simulink model "SiDLEngine"  (R2021a)
settings: Solver=VariableStepAuto  StartTime=0.0  StopTime=inf  FixedStep=0.03  RelTol=1e-3  EnableMultiTasking=on
model workspace (MAT data in the model file):
  AfrStoich = 14.6
  Cps = 2
  FuelSg = 0.75
  NCyl = 4
  Pstd = 101325
  Rair = 287
  TimeCnstECP = 0.01
  TimeCnstEGR = 0.01
  TimeCnstETC = 0.01
  TimeCnstICP = 0.01
  TimeCnstIVL = 0.125
  TimeCnstMFA = 0.125
  TimeCnstSWVA = 0.125
  TimeCnstVCR = 0.125
  TimeCnstVGT = 0.15
  TimeCnstVIRL = 0.125
  TimeCnstWGA = 0.01
  Ts = 0.01
  Tstd = 293.15
  Vd = 0.0015
  layer2Bias = [-0.102818198502 -0.0669189542532 -0.0175336152315 -0.0613032355905 -0.0570961982012 -0.061625469476 -0.0630445405841 -0.102546460927 -0.0423759259284 -0.0306564457715 -0.0652378797531 -0.129787817597 ... (800 elements, 800x1)]
  layer2InputWeights = [-0.0867959260941 0.0265881456435 -0.00261938013136 0.0648385435343 -0.0334306880832 -0.044301789254 0.0604524612427 0.00893297791481 -0.0994751527905 0.0255589019507 -0.122370123863 -0.0740034654737 ... (1600 elements, 800x2)]
  layer2RecurrentWeights = [-0.015235141851 -0.11403311789 0.112884886563 0.0588350631297 0.0682250186801 0.0444636531174 -0.0968889594078 -0.0397337339818 -0.0227067749947 0.0294026453048 -0.0304179247469 -0.145884677768 ... (160000 elements, 800x200)]
  layer3Bias = [0.0529259070754; 0.0636636316776; 0.0140457563102; 0.0780845806003; 0.0347621031106; -0.023198319599; -0.0368600413203; -0.00711429771036; -0.0257519558072; 0.0254531633109; 0.0144603000954]
  layer3Weights = [0.0566984564066 0.0242331400514 0.158808469772 0.0399505831301 -0.0030719502829 0.0837587192655 0.0579013302922 -0.0333247296512 -0.120384372771 -0.125806882977 0.0938690528274 -0.052338026464 ... (2200 elements, 11x200)]
  muX = [2220.83734119 107.92815484]
  muY = [104.671657967 115562.072489 0.00224719893222 986.056400633 7383.06398882 0.0299760704621 325.741103054 5.88867806863e-05 0.000942478781448 3.56158507349e-05 0.00543639293543]
  sigX = [1470.27383875 63.5647381428]
  sigY = [65.6275263528 46686.4071583 0.00207427504126 224.539922164 5111.0011239 0.0252132241042 8.06209455442 0.000125926264941 0.00171123843744 4.89959895827e-05 0.00480295587248]
libraries: autolibutils x4, simulink x2, autolibsharedmappedenginescommon x1, autolibpowerinfoutils x1
(part 1 of 2)
settings Model: ModifiedByFormat=The MathWorks, Inc.  OrderedModelArguments=off  Creator=The MathWorks, Inc.  LastModifiedBy=The MathWorks, Inc.
settings SolverCC: AlgebraicLoopSolver=TrustRegion  DecoupledContinuousIntegration=on
settings DataIOCC: DSMLogging=off  ReturnWorkspaceOutputs=off
settings DebuggingCC: SFMachineParentedDataDiag=warning  ArithmeticOperatorsInVariantConditions=warning
settings SFSimCC: SimUseLocalCustomCode=off
settings RTWCC: RTWUseLocalCustomCode=off
settings CodeAppCC: StateflowObjectComments=on
settings GRTTargetCC: TargetLangStandard=C89/C90 (ANSI)
settings ConfigComp: CovMetricSettings=dsw  CovSaveCumulativeToWorkspaceVar=on  CovSaveSingleToWorkspaceVar=on  CovExternalEMLEnable=off
settings SimscapeCC: SimscapeNormalizeSystem=off  SimscapeNominalValues={1, 'bar'; 1, 'cm^3/s'; 1, 'bar*kg/s'; 1, 'kJ/kg'; 1, 'kW'}

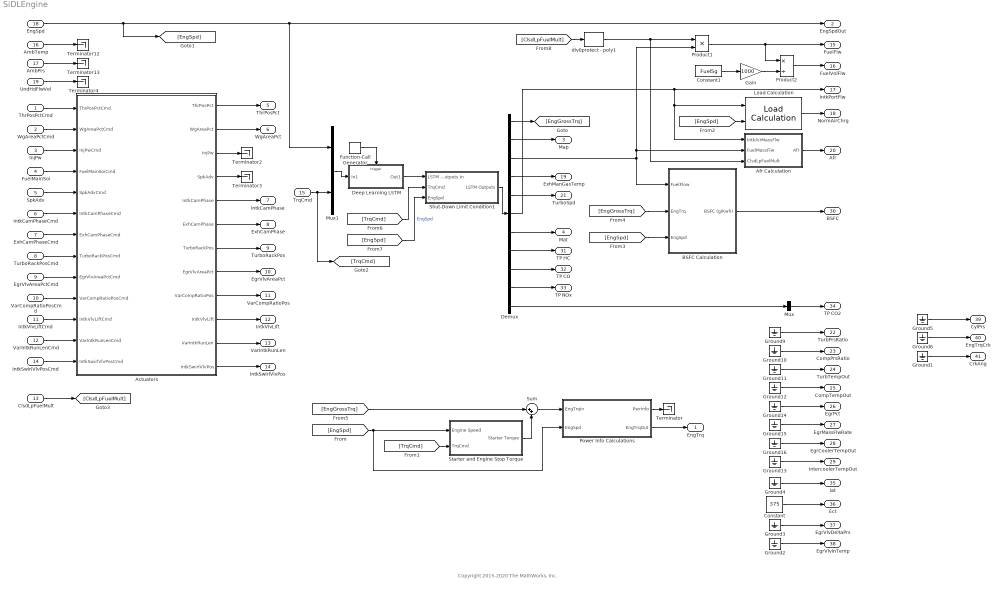
== system SiDLEngine ==
  note: Copyright 2015-2020 The MathWorks, Inc.
  ThrPosPctCmd : Inport
  WgAreaPctCmd : Inport  Port=2
  InjPw : Inport  Port=3
  FuelMainSoi : Inport  Port=4
  SpkAdv : Inport  Port=5
  IntkCamPhaseCmd : Inport  Port=6
  ExhCamPhaseCmd : Inport  Port=7
  TurboRackPosCmd : Inport  Port=8
  EgrVlvAreaPctCmd : Inport  Port=9
  VarCompRatioPosCmd : Inport  Port=10
  IntkVlvLiftCmd : Inport  Port=11
  VarIntkRunLenCmd : Inport  Port=12
  ClsdLpFuelMult : Inport  Port=13  Unit=1
  IntkSwirlVlvPosCmd : Inport  Port=14
  TrqCmd : Inport  Port=15  Unit=N*m
  AmbTemp : Inport  Port=16  Unit=K
  AmbPrs : Inport  Port=17  Unit=Pa
  EngSpd : Inport  Port=18  Interpolate=off
  UndHdFlwVel : Inport  Port=19  Unit=m/s
  Actuators : Subsystem
  Afr Calculation : Subsystem
  BSFC Calculation : Subsystem
  Constant : Constant  Value=375
  Constant1 : Constant  Value=FuelSg
  Deep Learning LSTM : Subsystem  TreatAsAtomicUnit=on
  Demux : Demux  Outputs=11
  Function-Call Generator : simulink/Ports & Subsystems/Function-Call Generator  sample_time=Ts  numberOfIterations=1  DisallowWideOutput=off
  Gain : Gain  Gain=1000
  Ground{1..6,9..16} (14 alike) : Ground
  Load Calculation : autolibsharedmappedenginescommon/Load Calculation  SystemSampleTime=-1  VariantActivationTime=update diagram  Latency=0  AutoFrameSizeCalculation=off
      settings: SourceProductBaseCode=PW,DR,MT,UV,VE
  Mux : Mux  Inputs=1
  Mux1 : Mux  Inputs=2
  Power Info Calculations : Subsystem
  Product1 : Product
  Product2 : Product  Inputs=*/
  Shut-Down Limit Condition1 : Subsystem
  Starter and Engine Stop Torque : Subsystem
  Sum : Sum  Inputs=|++
  Terminator{,2..4,12..13} (6 alike) : Terminator
  div0protect - poly1 : autolibutils/div0protect - poly  thresh=0.01  ZeroCross1=off  aMode=aMode
      settings: SourceProductBaseCode=PW,DR,MT,UV,VE
  EngTrq : Outport  Unit=N*m  VectorParamsAs1DForOutWhenUnconnected=off
  EngSpdOut : Outport  Port=2  VectorParamsAs1DForOutWhenUnconnected=off
  Map : Outport  Port=3  Unit=Pa  VectorParamsAs1DForOutWhenUnconnected=off
  Mat : Outport  Port=4  Unit=K  VectorParamsAs1DForOutWhenUnconnected=off
  ThrPosPct : Outport  Port=5  VectorParamsAs1DForOutWhenUnconnected=off
  WgAreaPct : Outport  Port=6  VectorParamsAs1DForOutWhenUnconnected=off
  IntkCamPhase : Outport  Port=7  VectorParamsAs1DForOutWhenUnconnected=off
  ExhCamPhase : Outport  Port=8  VectorParamsAs1DForOutWhenUnconnected=off
  TurboRackPos : Outport  Port=9  VectorParamsAs1DForOutWhenUnconnected=off
  EgrVlvAreaPct : Outport  Port=10  VectorParamsAs1DForOutWhenUnconnected=off
  VarCompRatioPos : Outport  Port=11  VectorParamsAs1DForOutWhenUnconnected=off
  IntkVlvLift : Outport  Port=12  VectorParamsAs1DForOutWhenUnconnected=off
  VarIntkRunLen : Outport  Port=13  VectorParamsAs1DForOutWhenUnconnected=off
  IntkSwirlVlvPos : Outport  Port=14  VectorParamsAs1DForOutWhenUnconnected=off
  FuelFlw : Outport  Port=15  Unit=kg/s  VectorParamsAs1DForOutWhenUnconnected=off
  FuelVolFlw : Outport  Port=16  Unit=m^3/s  VectorParamsAs1DForOutWhenUnconnected=off
  IntkPortFlw : Outport  Port=17  Unit=kg/s  VectorParamsAs1DForOutWhenUnconnected=off
  NormAirChrg : Outport  Port=18  Unit=1  VectorParamsAs1DForOutWhenUnconnected=off
  ExhManGasTemp : Outport  Port=19  Unit=K  VectorParamsAs1DForOutWhenUnconnected=off
  Afr : Outport  Port=20  Unit=1  VectorParamsAs1DForOutWhenUnconnected=off
  TurboSpd : Outport  Port=21  Unit=rad/s  VectorParamsAs1DForOutWhenUnconnected=off
  TurbPrsRatio : Outport  Port=22  Unit=1  VectorParamsAs1DForOutWhenUnconnected=off
  CompPrsRatio : Outport  Port=23  Unit=1  VectorParamsAs1DForOutWhenUnconnected=off
  TurbTempOut : Outport  Port=24  Unit=K  VectorParamsAs1DForOutWhenUnconnected=off
  CompTempOut : Outport  Port=25  Unit=K  VectorParamsAs1DForOutWhenUnconnected=off
  EgrPct : Outport  Port=26  Unit=%  VectorParamsAs1DForOutWhenUnconnected=off
  EgrMassFlwRate : Outport  Port=27  Unit=kg/s  VectorParamsAs1DForOutWhenUnconnected=off
  EgrCoolerTempOut : Outport  Port=28  Unit=K  VectorParamsAs1DForOutWhenUnconnected=off
  IntercoolerTempOut : Outport  Port=29  Unit=K  VectorParamsAs1DForOutWhenUnconnected=off
  BSFC : Outport  Port=30  Unit=g/(kW*hr)  VectorParamsAs1DForOutWhenUnconnected=off
  TP HC : Outport  Port=31  Unit=kg/s  VectorParamsAs1DForOutWhenUnconnected=off
  TP CO : Outport  Port=32  Unit=kg/s  VectorParamsAs1DForOutWhenUnconnected=off
  TP NOx : Outport  Port=33  Unit=kg/s  VectorParamsAs1DForOutWhenUnconnected=off
  TP CO2 : Outport  Port=34  Unit=kg/s  VectorParamsAs1DForOutWhenUnconnected=off
  Iat : Outport  Port=35  Unit=K  VectorParamsAs1DForOutWhenUnconnected=off
  Ect : Outport  Port=36  Unit=K  VectorParamsAs1DForOutWhenUnconnected=off
  EgrVlvDeltaPrs : Outport  Port=37  Unit=Pa  VectorParamsAs1DForOutWhenUnconnected=off
  EgrVlvInTemp : Outport  Port=38  Unit=K  VectorParamsAs1DForOutWhenUnconnected=off
  CylPrs : Outport  Port=39  VectorParamsAs1DForOutWhenUnconnected=off
  EngTrqCrk : Outport  Port=40  VectorParamsAs1DForOutWhenUnconnected=off
  CrkAng : Outport  Port=41  VectorParamsAs1DForOutWhenUnconnected=off
  wires:
  Demux/6 -> Load Calculation/1, Afr Calculation/1(IntkAirMassFlw), IntkPortFlw/1
  Demux/11 -> Mux/1
  Demux/9 -> TP CO/1
  Mux/1 -> TP CO2/1
  IntkCamPhaseCmd/1 -> Actuators/6(IntkCamPhaseCmd)
  Ground16/1 -> EgrCoolerTempOut/1
  Ground13/1 -> IntercoolerTempOut/1
  Ground12/1 -> CompTempOut/1
  FuelMainSoi/1 -> Actuators/4(FuelMainSoiCmd)
  EgrVlvAreaPctCmd/1 -> Actuators/9(EgrVlvAreaPctCmd)
  Ground11/1 -> TurbTempOut/1
  ExhCamPhaseCmd/1 -> Actuators/7(ExhCamPhaseCmd)
  Ground9/1 -> TurbPrsRatio/1
  SpkAdv/1 -> Actuators/5(SpkAdvCmd)
  AmbTemp/1 -> Terminator12/1
  Ground15/1 -> EgrMassFlwRate/1
  TurboRackPosCmd/1 -> Actuators/8(TurboRackPosCmd)
  ThrPosPctCmd/1 -> Actuators/1(ThrPosPctCmd)
  WgAreaPctCmd/1 -> Actuators/2(WgAreaPctCmd)
  InjPw/1 -> Actuators/3(InjPwCmd)
  Ground10/1 -> CompPrsRatio/1
  Demux/7 -> Mat/1
  Demux/2 -> Map/1
  AmbPrs/1 -> Terminator13/1
  IntkVlvLiftCmd/1 -> Actuators/11(IntkVlvLiftCmd)
  VarCompRatioPosCmd/1 -> Actuators/10(VarCompRatioPosCmd)
  VarIntkRunLenCmd/1 -> Actuators/12(VarIntkRunLenCmd)
  IntkSwirlVlvPosCmd/1 -> Actuators/13(IntkSwirlVlvPosCmd)
  UndHdFlwVel/1 -> Terminator4/1
  Actuators/5(IntkCamPhase) -> IntkCamPhase/1
  Actuators/6(ExhCamPhase) -> ExhCamPhase/1
  Actuators/7(TurboRackPos) -> TurboRackPos/1
  Actuators/8(EgrVlvAreaPct) -> EgrVlvAreaPct/1
  Actuators/9(VarCompRatioPos) -> VarCompRatioPos/1
  Actuators/10(IntkVlvLift) -> IntkVlvLift/1
  Actuators/11(VarIntkRunLen) -> VarIntkRunLen/1
  Actuators/12(IntkSwirlVlvPos) -> IntkSwirlVlvPos/1
  Constant/1 -> Ect/1
  Ground2/1 -> EgrVlvInTemp/1
  Ground3/1 -> EgrVlvDeltaPrs/1
  Ground4/1 -> Iat/1
  Power Info Calculations/1(PwrInfo) -> Terminator/1
  Demux/3 -> Afr Calculation/2(FuelMassFlw), Product1/2, BSFC Calculation/1(FuelFlow)
  Product2/1 -> FuelVolFlw/1
  ClsdLpFuelMult/1 -> [ClsdLpFuelMult]
  Deep Learning LSTM/1(Out1) -> Shut-Down Limit Condition1/1(LSTM Outputs In)
  Demux/4 -> ExhManGasTemp/1
  Demux/5 -> TurboSpd/1
  Constant1/1 -> Gain/1
  Starter and Engine Stop Torque/1(Starter Torque) -> Sum/2
  Sum/1 -> Power Info Calculations/1(EngTrqIn)
  Function-Call Generator/1 -> Deep Learning LSTM/Trigger
  Ground14/1 -> EgrPct/1
  Gain/1 -> Product2/2
  Power Info Calculations/2(EngTrqOut) -> EngTrq/1
  [EngSpd] -> Starter and Engine Stop Torque/1(Engine Speed), Power Info Calculations/2(EngSpd)
  Afr Calculation/1(Afr) -> Afr/1
  Load Calculation/1 -> NormAirChrg/1
  [EngSpd] -> Load Calculation/2
  BSFC Calculation/1(BSFC (g/Kwh)) -> BSFC/1
  [EngSpd] -> BSFC Calculation/3(EngSpd)
  [EngGrossTrq] -> BSFC Calculation/2(EngTrq)
  [TrqCmd] -> Starter and Engine Stop Torque/2(TrqCmd)
  Shut-Down Limit Condition1/1(LSTM Outputs) -> Demux/1
  [EngSpd] -> Shut-Down Limit Condition1/3(EngSpd)  "EngSpd"
  EngSpd/1 -> [EngSpd], Mux1/1, EngSpdOut/1
  Actuators/1(ThrPosPct) -> ThrPosPct/1
  Actuators/2(WgAreaPct) -> WgAreaPct/1
  Actuators/3(InjPw) -> Terminator2/1
  Actuators/4(SpkAdv) -> Terminator3/1
  [EngGrossTrq] -> Sum/1
  Mux1/1 -> Deep Learning LSTM/1(In1)
  Demux/1 -> [EngGrossTrq]
  TrqCmd/1 -> [TrqCmd], Mux1/2
  Demux/8 -> TP HC/1
  Demux/10 -> TP NOx/1
  [TrqCmd] -> Shut-Down Limit Condition1/2(TrqCmd)
  [ClsdLpFuelMult] -> div0protect - poly1/1
  Product1/1 -> Product2/1, FuelFlw/1
  div0protect - poly1/1 -> Afr Calculation/3(ClsdLpFuelMult), Product1/1
  Ground5/1 -> CylPrs/1
  Ground6/1 -> EngTrqCrk/1
  Ground1/1 -> CrkAng/1
